simulink model "Compare_lin_nonlin"  (R2019b)
settings: Solver=VariableStepAuto  StartTime=0.0  StopTime=6  RelTol=1e-3
settings Model: Creator=cambr  LastModifiedBy=cambr

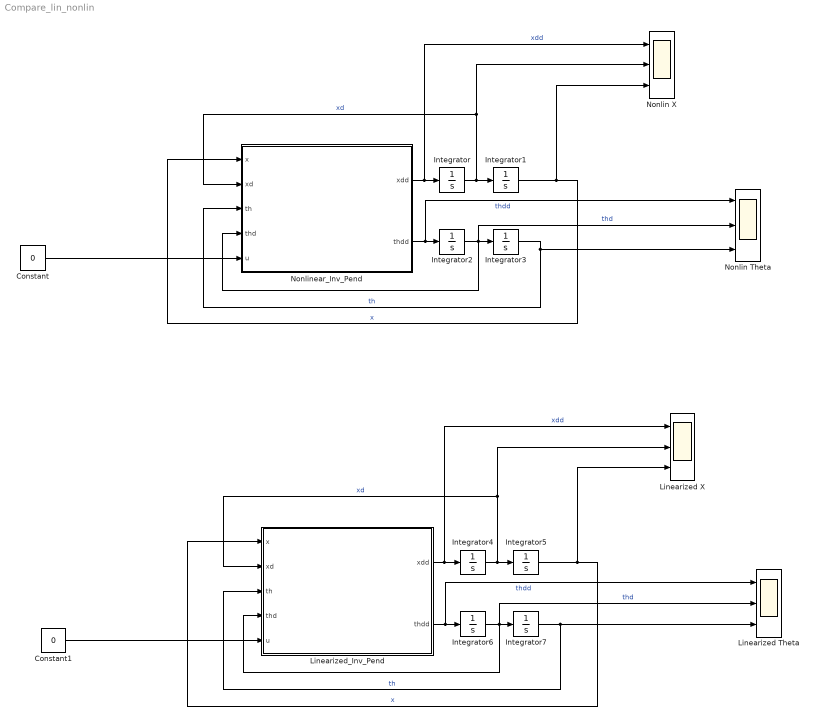
== system Compare_lin_nonlin ==
  Constant : Constant  Value=0
  Constant1 : Constant  Value=0
  Integrator{,1..2,4..6} (6 alike) : Integrator
  Integrator3 : Integrator  InitialCondition=0.01
  Integrator7 : Integrator  InitialCondition=0.01
  Linearized Theta : Scope  NumInputPorts=3
  Linearized X : Scope  NumInputPorts=3
  Linearized_Inv_Pend : MATLAB Function  TreatAsAtomicUnit=on
  Nonlin Theta : Scope  NumInputPorts=3
  Nonlin X : Scope  NumInputPorts=3
  Nonlinear_Inv_Pend : MATLAB Function  TreatAsAtomicUnit=on
  wires:
  Integrator/1 -> Integrator1/1, Nonlin X/2, Nonlinear_Inv_Pend/2(xd)  "xd"
  Integrator1/1 -> Nonlin X/3, Nonlinear_Inv_Pend/1(x)  "x"
  Nonlinear_Inv_Pend/1(xdd) -> Nonlin X/1, Integrator/1  "xdd"
  Integrator3/1 -> Nonlinear_Inv_Pend/3(th), Nonlin Theta/3  "th"
  Integrator2/1 -> Nonlin Theta/2, Integrator3/1, Nonlinear_Inv_Pend/4(thd)  "thd"
  Nonlinear_Inv_Pend/2(thdd) -> Nonlin Theta/1, Integrator2/1  "thdd"
  Constant/1 -> Nonlinear_Inv_Pend/5(u)
  Integrator5/1 -> Linearized X/3, Linearized_Inv_Pend/1(x)  "x"
  Linearized_Inv_Pend/2(thdd) -> Linearized Theta/1, Integrator6/1  "thdd"
  Constant1/1 -> Linearized_Inv_Pend/5(u)
  Integrator6/1 -> Linearized Theta/2, Integrator7/1, Linearized_Inv_Pend/4(thd)  "thd"
  Integrator7/1 -> Linearized_Inv_Pend/3(th), Linearized Theta/3  "th"
  Linearized_Inv_Pend/1(xdd) -> Linearized X/1, Integrator4/1  "xdd"
  Integrator4/1 -> Integrator5/1, Linearized X/2, Linearized_Inv_Pend/2(xd)  "xd"

== matlab function Compare_lin_nonlin/Linearized_Inv_Pend ==
  data: x input size=1; xd input size=1; xdd output size=1; thdd output size=1; th input size=1; thd input size=1; u input
function [xdd, thdd] = fcn(x, xd, th, thd, u)

g = 9.8; % gravity
m = 0.08; % kg, pendulum mass, meas 0.08
M = 0.32; % kg, cart mass, meas 0.32
l = 0.17; % meters, center of mass location on pendulum, meas 0.17
I = 3.5e-3; %1/3*m1*r^2 + m2*L^2;, meas 3.5e-3
b = 0.01; % N/(m/s)

xdd = (u - m*g*th)/(M);
thdd = (u -(M+m)*g*th)/(-M*l);

== matlab function Compare_lin_nonlin/Nonlinear_Inv_Pend ==
  data: x input size=1; xd input size=1; xdd output size=1; thdd output size=1; th input size=1; thd input size=1; u input
function [xdd, thdd] = fcn(x, xd, th, thd, u)

g = 9.8; % gravity
m = 0.08; % kg, pendulum mass, meas 0.08
M = 0.32; % kg, cart mass, meas 0.32
l = 0.17; % meters, center of mass location on pendulum, meas 0.17
I = 3.5e-3; %1/3*m1*r^2 + m2*L^2;, meas 3.5e-3
b = 0.01; % N/(m/s)

xdd = (u + m*l*sin(th)*thd^2 - m*g*cos(th)*sin(th))/(M + m - m*cos(th)^2);
thdd = (u*cos(th) - (M+m)*g*sin(th) + m*l*cos(th)*sin(th)*thd^2)/(m*l*cos(th)^2 - (M+m)*l);
